simulink model "readEncoder"  (R2022a)
settings: Solver=FixedStepAuto  StartTime=0.0  StopTime=inf  FixedStep=0.01  RelTol=1e-3  EnableMultiTasking=on
undefined symbols (not defined in the file): a, b, c1, c2, g, J2, K, Kb, Kt, Ra, theta_0
libraries: simulink_extras x3
settings Model: ExtModeTrigDuration=10  Creator=adlipke  LastModifiedBy=adlipke
settings OptimizationCC: EnhancedBackFolding=on  PassReuseOutputArgsAs=Individual arguments  ZeroExternalMemoryAtStartup=off  ZeroInternalMemoryAtStartup=off  MaxStackSize=64  OptimizeBlockOrder=speed  DifferentSizesBufferReuse=on  OptimizationCustomize=off  EfficientTunableParamExpr=on
settings DebuggingCC: InheritedTsInSrcMsg=none  ParameterTunabilityLossMsg=error
settings HardwareCC: ProdBitPerPointer=32  ProdBitPerSizeT=32  ProdBitPerPtrDiffT=32  ProdLargestAtomicInteger=Long  ProdLargestAtomicFloat=Double  ProdWordSize=32  ProdLongLongMode=on  ProdHWDeviceType=ARM Compatible->ARM Cortex
settings SFSimCC: MATLABDynamicMemAlloc=off
settings RTWCC: SystemTargetFile=ert.tlc  HardwareBoard=STM32 Nucleo L476RG  TemplateMakefile=ert_default_tmf  Toolchain=GNU Tools for ARM Embedded Processors
settings CodeAppCC: ForceParamTrailComments=on  IgnoreCustomStorageClasses=off  OperatorAnnotations=on  SimulinkDataObjDesc=on  SFDataObjDesc=on  InsertBlockDesc=on
settings ERTTargetCC: ExtModeTransport=3  ExtModeStaticAlloc=on  ExtModeStaticAllocSize=2000  ExtModeMexFile=ext_xcp  ExtModeIntrfLevel=Level2 - Open

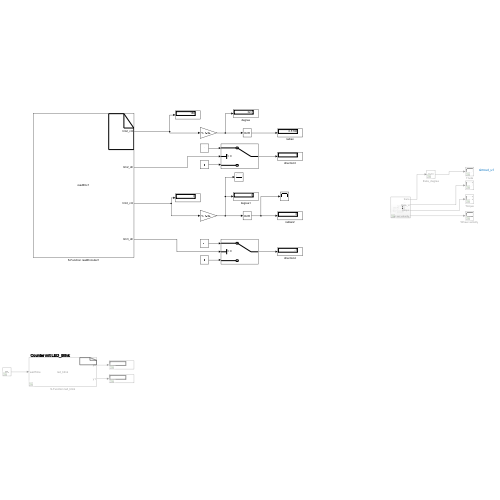
[thumbnail: Simulink's stored preview of the top-level diagram]
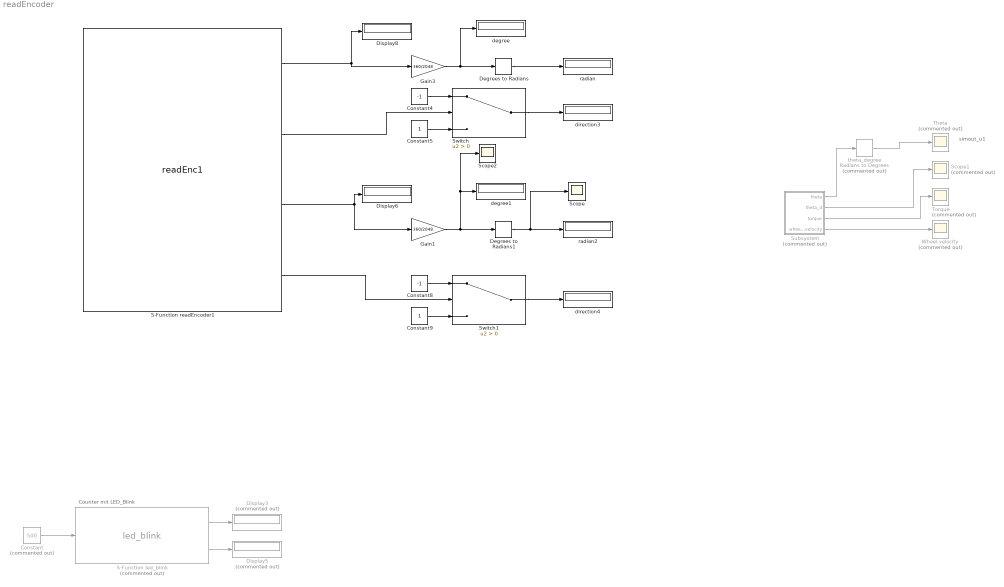
== system readEncoder ==
  note: Counter mit LED_Blink
  note: simout_u1
  Constant : Constant  Commented=on  Value=500
  Constant4 : Constant  Value=-1
  Constant5 : Constant
  Constant8 : Constant  Value=-1
  Constant9 : Constant
  Degrees to Radians : simulink_extras/Transformations/Degrees to Radians
  Degrees to Radians1 : simulink_extras/Transformations/Degrees to Radians
  Display3 : Display  Commented=on
  Display5 : Display  Commented=on
  Display6 : Display
  Display8 : Display
  Gain1 : Gain  Gain=360/2048
  Gain3 : Gain  Gain=360/2048
  S-Function led_blink : S-Function  Commented=on  FunctionName=led_blink  SFunctionModules=led_blink_wrapper  SFunctionDeploymentMode=off  EnableBusSupport=off  mask(S-Function Builder){}
      mask help: Simulink:masks:SFunctionBuilder_MD
      mask init:
      | val = [[.9  0.75 0.75 1 1 .9 .9 1]',[1 1 0.75 0.75 .9 .9 1 .9]'];try , sys = get_param(gcb,'SfunBuilderFcnName');if isempty(sys), sys = get_param(gcb,'FunctionName'); end,catch, sys = get_param(gcb,'FunctionName'); end
      settings: CopyFcn=set_param(gcbh,'LinkStatus','none')  OpenFcn=sfunctionwizard(gcbh)
      mask Display:
      | plot(val(:,1),val(:,2))
      | disp(sys)
      | port_label('input',1,'waitTime')
      | port_label('output',1,'y0')
      | port_label('output',2,'y1')
  S-Function readEncoder1 : S-Function  FunctionName=readEnc1  SFunctionModules=readEnc1_wrapper  SFunctionDeploymentMode=off  EnableBusSupport=off  mask(S-Function Builder){}
      mask help: Simulink:masks:SFunctionBuilder_MD
      mask init: same as readEncoder/S-Function led_blink
      settings: CopyFcn=set_param(gcbh,'LinkStatus','none')  OpenFcn=sfunctionwizard(gcbh)
      mask Display:
      | plot(val(:,1),val(:,2))
      | disp(sys)
      | port_label('output',1,'tim2_cnt')
      | port_label('output',2,'tim2_dir')
      | port_label('output',3,'tim3_cnt')
      | port_label('output',4,'tim3_dir')
  Scope : Scope
  Scope1 : Scope  Commented=on
  Scope2 : Scope
  Subsystem : Subsystem  Commented=on
  Switch : Switch  Criteria=u2 > Threshold  SaturateOnIntegerOverflow=off  InputSameDT=off
  Switch1 : Switch  Criteria=u2 > Threshold  SaturateOnIntegerOverflow=off  InputSameDT=off
  Theta : Scope  Commented=on
  Torque : Scope  Commented=on
  Wheel velocity : Scope  Commented=on
  degree : Display
  degree1 : Display
  direction3 : Display
  direction4 : Display
  radian : Display
  radian2 : Display
  theta_degree : simulink_extras/Transformations/Radians to Degrees  Commented=on
  wires:
  S-Function led_blink/1 -> Display3/1
  Constant/1 -> S-Function led_blink/1
  S-Function led_blink/2 -> Display5/1
  Gain3/1 -> degree/1, Degrees to Radians/1
  Constant9/1 -> Switch1/3
  S-Function readEncoder1/4 -> Switch1/2
  Degrees to Radians1/1 -> Scope/1, radian2/1
  Switch/1 -> direction3/1
  Constant8/1 -> Switch1/1
  S-Function readEncoder1/2 -> Switch/2
  S-Function readEncoder1/1 -> Gain3/1, Display8/1
  S-Function readEncoder1/3 -> Gain1/1, Display6/1
  Gain1/1 -> Degrees to Radians1/1, Scope2/1, degree1/1
  Constant4/1 -> Switch/1
  Switch1/1 -> direction4/1
  Degrees to Radians/1 -> radian/1
  Constant5/1 -> Switch/3
  Subsystem/3(torque) -> Torque/1
  Subsystem/4(wheel velocity) -> Wheel velocity/1
  Subsystem/1(theta) -> theta_degree/1
  theta_degree/1 -> Theta/1
  Subsystem/2(theta_d) -> Scope1/1

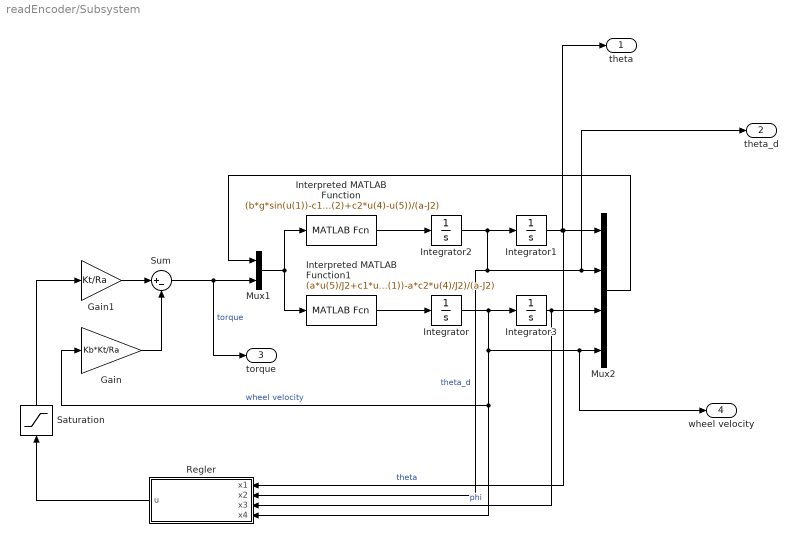
== system readEncoder/Subsystem ==
  Gain : Gain  Gain=Kb*Kt/Ra
  Gain1 : Gain  Gain=Kt/Ra
  Integrator : Integrator
  Integrator1 : Integrator  InitialCondition=theta_0
  Integrator2 : Integrator
  Integrator3 : Integrator
  Interpreted MATLAB Function : MATLABFcn  MATLABFcn=(b*g*sin(u(1))-c1*u(2)+c2*u(4)-u(5))/(a-J2)  Output1D=off
  Interpreted MATLAB Function1 : MATLABFcn  MATLABFcn=(a*u(5)/J2+c1*u(2)-b*g*sin(u(1))-a*c2*u(4)/J2)/(a-J2)  Output1D=off
  Mux1 : Mux  Inputs=2
  Mux2 : Mux
  Regler : Subsystem
  Saturation : Saturate  UpperLimit=30  LowerLimit=-30
  Sum : Sum  Inputs=|+-
  theta : Outport
  theta_d : Outport  Port=2
  torque : Outport  Port=3
  wheel velocity : Outport  Port=4
  wires:
  Integrator1/1 -> theta/1, Mux2/1, Regler/1(x1)  "theta"
  Integrator2/1 -> Integrator1/1, Regler/2(x2), theta_d/1, Mux2/2  "theta_d"
  Integrator3/1 -> Regler/3(x3), Mux2/3  "phi"
  Gain/1 -> Sum/2
  Mux2/1 -> Mux1/1
  Sum/1 -> torque/1, Mux1/2  "torque"
  Integrator/1 -> Regler/4(x4), Gain/1, wheel velocity/1, Mux2/4, Integrator3/1  "wheel velocity"
  Interpreted MATLAB Function/1 -> Integrator2/1
  Interpreted MATLAB Function1/1 -> Integrator/1
  Regler/1(u) -> Saturation/1
  Gain1/1 -> Sum/1
  Mux1/1 -> Interpreted MATLAB Function1/1, Interpreted MATLAB Function/1
  Saturation/1 -> Gain1/1

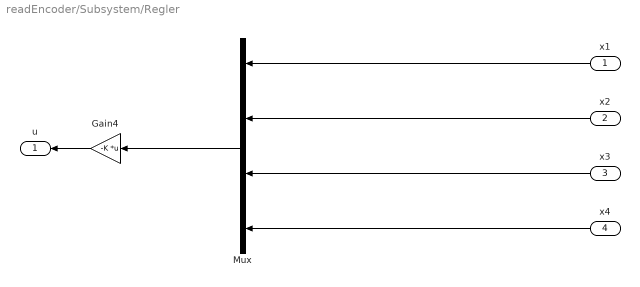
== system readEncoder/Subsystem/Regler ==
  x1 : Inport
  x2 : Inport  Port=2
  x3 : Inport  Port=3
  x4 : Inport  Port=4
  Gain4 : Gain  Gain=-K  Multiplication=Matrix(K*u)
  Mux : Mux
  u : Outport
  wires:
  Mux/1 -> Gain4/1
  Gain4/1 -> u/1
  x1/1 -> Mux/1
  x2/1 -> Mux/2
  x3/1 -> Mux/3
  x4/1 -> Mux/4
